simulink model "DOUBLESUPLMsim"  (R2022b)
settings: Solver=VariableStepAuto  StartTime=0.0  StopTime=10.0  RelTol=1e-3
libraries: fl_lib x27, nesl_utility x3
settings Model: Creator=andre.pianca  LastModifiedBy=andre.pianca

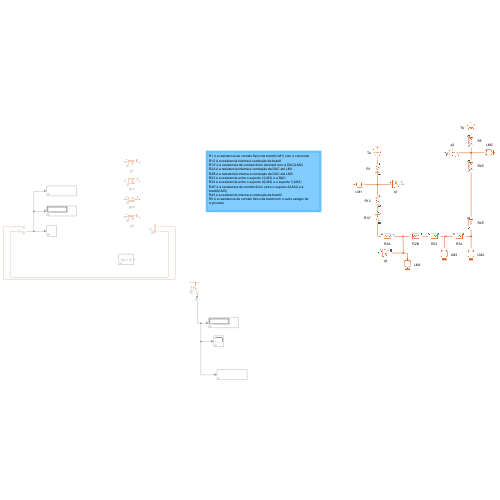
[thumbnail: Simulink's stored preview of the top-level diagram]
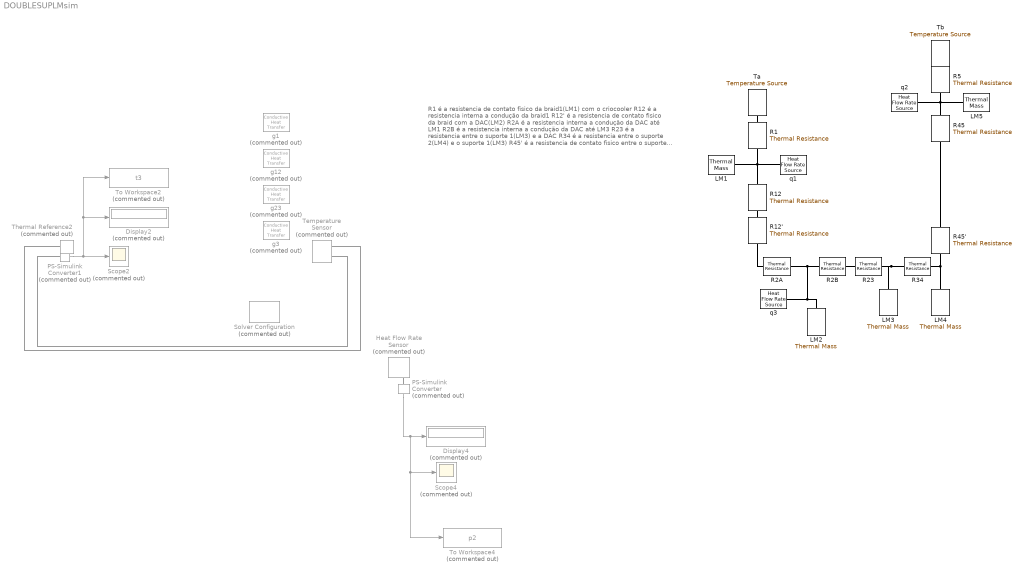
== system DOUBLESUPLMsim ==
  note: R1 é a resistencia de contato fisico da braid1(LM1) com o criocooler
      | R12 é a resistencia interna a condução da braid1
      | R12' é a resistencia de contato fisico da braid com a DAC(LM2)
      | R2A é a resistencia interna a condução da DAC até LM1
      | R2B é a resistencia interna a condução da DAC até LM3
      | R23 é a resistencia entre o suporte 1(LM3) e a DAC
      | R34 é a resistencia entre o suporte 2(LM4) e o suporte 1(LM3)
      | R45' é a resistencia de contato fisico entre o suporte 2(LM4) e a braid2(LM5)
      | R45 é a resistencia interna a condução da braid2
      | R5 é a resistencia de contato fisico da braid com o outro estagio do cryocooler
  Display2 : Display  Commented=on
  Display4 : Display  Commented=on
  Heat Flow Rate Sensor : fl_lib/Thermal/Thermal Sensors/Heat Flow Rate Sensor  Commented=on
  LM1 : fl_lib/Thermal/Thermal Elements/Thermal Mass  mass=0.432 kg  sp_heat=295.3784090389102 J/(K*kg)  num_ports=foundation.enum.numPorts2.one  T_specify=on  T_priority=None  T=300 K  T_nominal_specify=off  T_nominal_unit=K  T_nominal_value=1  Q_specify=off  Q_priority=None  Q=0 W  Q_nominal_specify=off  Q_nominal_unit=W  Q_nominal_value=1
  LM2 : fl_lib/Thermal/Thermal Elements/Thermal Mass  mass=0.432 kg  sp_heat=295.3784090389102 J/(K*kg)  num_ports=foundation.enum.numPorts2.one  T_specify=on  T_priority=None  T=300 K  T_nominal_specify=off  T_nominal_unit=K  T_nominal_value=1  Q_specify=off  Q_priority=None  Q=0 W  Q_nominal_specify=off  Q_nominal_unit=W  Q_nominal_value=1
  LM3 : fl_lib/Thermal/Thermal Elements/Thermal Mass  mass=0.332 kg  sp_heat=351.62703271694176 J/(K*kg)  num_ports=foundation.enum.numPorts2.one  T_specify=on  T_priority=None  T=300 K  T_nominal_specify=off  T_nominal_unit=K  T_nominal_value=1  Q_specify=off  Q_priority=None  Q=0 W  Q_nominal_specify=off  Q_nominal_unit=W  Q_nominal_value=1
  LM4 : fl_lib/Thermal/Thermal Elements/Thermal Mass  mass=0.332 kg  sp_heat=351.62703271694176 J/(K*kg)  num_ports=foundation.enum.numPorts2.one  T_specify=on  T_priority=None  T=300 K  T_nominal_specify=off  T_nominal_unit=K  T_nominal_value=1  Q_specify=off  Q_priority=None  Q=0 W  Q_nominal_specify=off  Q_nominal_unit=W  Q_nominal_value=1
  LM5 : fl_lib/Thermal/Thermal Elements/Thermal Mass  mass=0.332 kg  sp_heat=351.62703271694176 J/(K*kg)  num_ports=foundation.enum.numPorts2.one  T_specify=on  T_priority=None  T=300 K  T_nominal_specify=off  T_nominal_unit=K  T_nominal_value=1  Q_specify=off  Q_priority=None  Q=0 W  Q_nominal_specify=off  Q_nominal_unit=W  Q_nominal_value=1
  PS-Simulink Converter : nesl_utility/PS-Simulink Converter  Commented=on  PhysicalDomain=network_engine_domain  SubClassName=ps_output  LeftPortType=input  RightPortType=output  PseudoPeriodic=off  Frequencies=[]  VectorFormat=inherit  Unit=inherit  AffineConversion=off
  PS-Simulink Converter1 : nesl_utility/PS-Simulink Converter  Commented=on  PhysicalDomain=network_engine_domain  SubClassName=ps_output  LeftPortType=input  RightPortType=output  PseudoPeriodic=off  Frequencies=[]  VectorFormat=inherit  Unit=inherit  AffineConversion=off
  R{1,5,34,45} (4 alike) : fl_lib/Thermal/Thermal Elements/Thermal Resistance  resistance=1 K/W  T_specify=off  T_priority=None  T=0 K  T_nominal_specify=off  T_nominal_unit=K  T_nominal_value=1  Q_specify=off  Q_priority=None  Q=0 W  Q_nominal_specify=off  Q_nominal_unit=W  Q_nominal_value=1
  R12 : fl_lib/Thermal/Thermal Elements/Thermal Resistance  resistance=100000 K/W  T_specify=off  T_priority=None  T=0 K  T_nominal_specify=off  T_nominal_unit=K  T_nominal_value=1  Q_specify=off  Q_priority=None  Q=0 W  Q_nominal_specify=off  Q_nominal_unit=W  Q_nominal_value=1
  R12' : fl_lib/Thermal/Thermal Elements/Thermal Resistance  resistance=100000 K/W  T_specify=off  T_priority=None  T=0 K  T_nominal_specify=off  T_nominal_unit=K  T_nominal_value=1  Q_specify=off  Q_priority=None  Q=0 W  Q_nominal_specify=off  Q_nominal_unit=W  Q_nominal_value=1
  R23 : fl_lib/Thermal/Thermal Elements/Thermal Resistance  resistance=100000 K/W  T_specify=off  T_priority=None  T=0 K  T_nominal_specify=off  T_nominal_unit=K  T_nominal_value=1  Q_specify=off  Q_priority=None  Q=0 W  Q_nominal_specify=off  Q_nominal_unit=W  Q_nominal_value=1
  R2A : fl_lib/Thermal/Thermal Elements/Thermal Resistance  resistance=100000 K/W  T_specify=off  T_priority=None  T=0 K  T_nominal_specify=off  T_nominal_unit=K  T_nominal_value=1  Q_specify=off  Q_priority=None  Q=0 W  Q_nominal_specify=off  Q_nominal_unit=W  Q_nominal_value=1
  R2B : fl_lib/Thermal/Thermal Elements/Thermal Resistance  resistance=100000 K/W  T_specify=off  T_priority=None  T=0 K  T_nominal_specify=off  T_nominal_unit=K  T_nominal_value=1  Q_specify=off  Q_priority=None  Q=0 W  Q_nominal_specify=off  Q_nominal_unit=W  Q_nominal_value=1
  R45' : fl_lib/Thermal/Thermal Elements/Thermal Resistance  resistance=1 K/W  T_specify=off  T_priority=None  T=0 K  T_nominal_specify=off  T_nominal_unit=K  T_nominal_value=1  Q_specify=off  Q_priority=None  Q=0 W  Q_nominal_specify=off  Q_nominal_unit=W  Q_nominal_value=1
  Scope2 : Scope  Commented=on
  Scope4 : Scope  Commented=on
  Solver Configuration : nesl_utility/Solver Configuration  Commented=on  PhysicalDomain=network_engine_domain  SubClassName=solver  LeftPortType=input  RightPortType=generic  Tones=[]  Harmonics=[]  SimulateNoise=off  Profile=off  UseLocalSampling=off  EnableSwitchedLinearOptims=on  FrequencyDomain=off  UseCCode=off  RelTol=0.001  AbsTol=0.001  MinStep=1e-09  ToWorkspace=off  RevertToSquareIcSolve=off  NumHomotopyIterations=100  PhasorMode=off  PhasorModeNumHarmonics=1  ConsistencySolver=NEWTON_XTOL_AFTER_FTOL  IndexReductionMethod=DerivativeReplacement  DoDC=off  ResidualTolerance=1e-09  ConsistencyTolSource=GLOBAL  ConsistencyAbsTol=0.001  ConsistencyRelTol=0.001  ConsistencyTolFactor=0.001  UseLocalSolver=off  LocalSolverChoice=NE_BACKWARD_EULER_ADVANCER  ResolveIndetEquations=on  FunctionEvalNumThread=1  LocalSolverSampleTime=0.001  DoFixedCost=off  MaxNonlinIter=3  MaxModeIter=2  ComputeImpulses=off  ImpulseIterations=2  LinearAlgebra=auto  LinearAlgebraNumThread=0  EquationFormulation=NE_TIME_EF  DelaysMemoryBudget=1024  AutomaticFiltering=on  FilteringTimeConstant=0.001  PartitionStorageMethod=AS_NEEDED  PartitionMemoryBudget=1024  PartitionMethod=ROBUST
  Ta : fl_lib/Thermal/Thermal Sources/Temperature Source  temperature=4.2 K
  Tb : fl_lib/Thermal/Thermal Sources/Temperature Source  temperature=40 K
  Temperature Sensor : fl_lib/Thermal/Thermal Sensors/Temperature Sensor  Commented=on
  Thermal Reference2 : fl_lib/Thermal/Thermal Elements/Thermal Reference  Commented=on
  To Workspace2 : ToWorkspace  Commented=on  VariableName=t3  SampleTime=-1
  To Workspace4 : ToWorkspace  Commented=on  VariableName=p2  SampleTime=-1
  g{1,3,12,23} (4 alike) : fl_lib/Thermal/Thermal Elements/Conductive Heat Transfer  Commented=on  thermal_type=foundation.enum.ConstantVariableTabulated.Constant  wall_geometry=foundation.enum.ConductionWallGeometry.Planar  area=1e-4 m^2  thickness=0.1 m  d_in=0.05 m  d_out=0.1 m  L=1 m  th_cond_min=10 W/(K*m)  th_cond=401 W/(K*m)  th_cond_TLU=[413, 401, 392, 383, 371, 357, 342] W/(K*m)  temp_TLU=[200, 273, 400, 600, 800, 1000, 1200] K  T_specify=off  T_priority=None  T=0 K  T_nominal_specify=off  T_nominal_unit=K  T_nominal_value=1  Q_specify=off  Q_priority=None  Q=0 W  Q_nominal_specify=off  Q_nominal_unit=W  Q_nominal_value=1
  q1 : fl_lib/Thermal/Thermal Sources/Heat Flow Rate Source  heat_flow=10e-3 W
      settings: InternalSimscapePortConfiguration="{\"Bottom\":[],\"Left\":[{\"id\":\"B\",\"label\":\"B\",\"type\":\"foundation.thermal.thermal\"}],\"Right\":[{\"id\":\"A\",\"label\":\"A\",\"type\":\"foundation.thermal.thermal\"}],\"Top\":[]}"
  q2 : fl_lib/Thermal/Thermal Sources/Heat Flow Rate Source  heat_flow=10e-3 W
      settings: InternalSimscapePortConfiguration="{\"Bottom\":[],\"Left\":[{\"id\":\"B\",\"label\":\"B\",\"type\":\"foundation.thermal.thermal\"}],\"Right\":[{\"id\":\"A\",\"label\":\"A\",\"type\":\"foundation.thermal.thermal\"}],\"Top\":[]}"
  q3 : fl_lib/Thermal/Thermal Sources/Heat Flow Rate Source  heat_flow=10e-3 W
      settings: InternalSimscapePortConfiguration="{\"Bottom\":[],\"Left\":[{\"id\":\"B\",\"label\":\"B\",\"type\":\"foundation.thermal.thermal\"}],\"Right\":[{\"id\":\"A\",\"label\":\"A\",\"type\":\"foundation.thermal.thermal\"}],\"Top\":[]}"
  wires:
  PS-Simulink Converter/1 -> To Workspace4/1, Scope4/1, Display4/1
  PS-Simulink Converter1/1 -> To Workspace2/1, Display2/1, Scope2/1
  connections:
  R1/LConn1 -- Ta/LConn1
  R23/RConn1 -- LM3/LConn1 -- R34/LConn1
  R23/LConn1 -- R2B/RConn1
  R45/LConn1 -- R45'/RConn1
  PS-Simulink Converter/LConn1 -- Heat Flow Rate Sensor/RConn1
  PS-Simulink Converter1/LConn1 -- Temperature Sensor/RConn2
  Thermal Reference2/LConn1 -- Temperature Sensor/RConn1
  R12/LConn1 -- q1/RConn1 -- R1/RConn1 -- LM1/LConn1
  LM5/LConn1 -- R45/RConn1 -- q2/RConn1 -- R5/LConn1
  R5/RConn1 -- Tb/LConn1
  R12/RConn1 -- R12'/LConn1
  R12'/RConn1 -- R2A/LConn1
  R45'/LConn1 -- LM4/LConn1 -- R34/RConn1
  R2B/LConn1 -- LM2/LConn1 -- q3/LConn1 -- R2A/RConn1
